simulink model "system_integration_v3"  (R2024a)
settings: Solver=FixedStepDiscrete  StartTime=0.0  StopTime=200  RelTol=1e-3
values from neighbouring files (symbols this model uses):
  Ts = 1/Fs    (= 7.50007500075e-06)    [new_generation_coeff.m]    (also in simon_test.m; simple_fft_test.m = 1/F; testPSD_c2d.m; testPSD_simulink.m)
undefined symbols (not defined in the file or in its folder): magnitude
libraries: hdlsllib x84, embmathops x6, hdlmdlgenlib x1, dsphdlxfrm2 x1
(part 3 of 5)

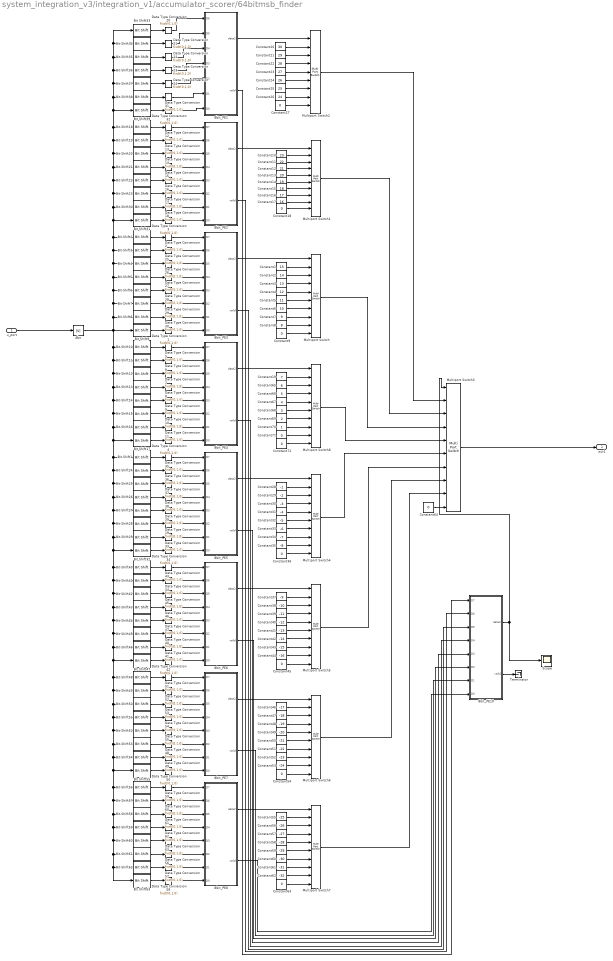
== system system_integration_v3/integration_v1/accumulator_scorer/64bitmsb_finder ==
  u_port : Inport
  8bit_PE1 : Subsystem
  8bit_PE10 : Subsystem
  8bit_PE2 : Subsystem
  8bit_PE3 : Subsystem
  8bit_PE4 : Subsystem
  8bit_PE5 : Subsystem
  8bit_PE6 : Subsystem
  8bit_PE7 : Subsystem
  8bit_PE8 : Subsystem
  Abs : Abs  SaturateOnIntegerOverflow=off
  Bit Shift1 : hdlsllib/Logic and Bit Operations/Bit Shift  mode=Shift Left Logical  N=1
  Bit Shift10 : hdlsllib/Logic and Bit Operations/Bit Shift  mode=Shift Right Logical  N=7
  Bit Shift11 : hdlsllib/Logic and Bit Operations/Bit Shift  mode=Shift Right Logical  N=6
  Bit Shift12 : hdlsllib/Logic and Bit Operations/Bit Shift  mode=Shift Right Logical  N=5
  Bit Shift13 : hdlsllib/Logic and Bit Operations/Bit Shift  mode=Shift Right Logical  N=4
  Bit Shift14 : hdlsllib/Logic and Bit Operations/Bit Shift  mode=Shift Right Logical  N=3
  Bit Shift15 : hdlsllib/Logic and Bit Operations/Bit Shift  mode=Shift Right Logical  N=2
  Bit Shift16 : hdlsllib/Logic and Bit Operations/Bit Shift  mode=Shift Right Logical  N=1
  Bit Shift17 : hdlsllib/Logic and Bit Operations/Bit Shift  mode=Shift Right Logical  N=0
  Bit Shift18 : hdlsllib/Logic and Bit Operations/Bit Shift  mode=Shift Right Logical  N=23
  Bit Shift19 : hdlsllib/Logic and Bit Operations/Bit Shift  mode=Shift Right Logical  N=22
  Bit Shift2 : hdlsllib/Logic and Bit Operations/Bit Shift  mode=Shift Right Logical  N=15
  Bit Shift20 : hdlsllib/Logic and Bit Operations/Bit Shift  mode=Shift Right Logical  N=21
  Bit Shift21 : hdlsllib/Logic and Bit Operations/Bit Shift  mode=Shift Right Logical  N=20
  Bit Shift22 : hdlsllib/Logic and Bit Operations/Bit Shift  mode=Shift Right Logical  N=19
  Bit Shift23 : hdlsllib/Logic and Bit Operations/Bit Shift  mode=Shift Right Logical  N=18
  Bit Shift24 : hdlsllib/Logic and Bit Operations/Bit Shift  mode=Shift Left Logical  N=2
  Bit Shift25 : hdlsllib/Logic and Bit Operations/Bit Shift  mode=Shift Left Logical  N=3
  Bit Shift26 : hdlsllib/Logic and Bit Operations/Bit Shift  mode=Shift Left Logical  N=4
  Bit Shift27 : hdlsllib/Logic and Bit Operations/Bit Shift  mode=Shift Left Logical  N=5
  Bit Shift28 : hdlsllib/Logic and Bit Operations/Bit Shift  mode=Shift Left Logical  N=6
  Bit Shift29 : hdlsllib/Logic and Bit Operations/Bit Shift  mode=Shift Left Logical  N=7
  Bit Shift3 : hdlsllib/Logic and Bit Operations/Bit Shift  mode=Shift Right Logical  N=14
  Bit Shift30 : hdlsllib/Logic and Bit Operations/Bit Shift  mode=Shift Right Logical  N=17
  Bit Shift31 : hdlsllib/Logic and Bit Operations/Bit Shift  mode=Shift Right Logical  N=16
  Bit Shift32 : hdlsllib/Logic and Bit Operations/Bit Shift  mode=Shift Left Logical  N=8
  Bit Shift33 : hdlsllib/Logic and Bit Operations/Bit Shift  mode=Shift Right Logical  N=30
  Bit Shift34 : hdlsllib/Logic and Bit Operations/Bit Shift  mode=Shift Right Logical  N=29
  Bit Shift35 : hdlsllib/Logic and Bit Operations/Bit Shift  mode=Shift Right Logical  N=28
  Bit Shift36 : hdlsllib/Logic and Bit Operations/Bit Shift  mode=Shift Right Logical  N=27
  Bit Shift37 : hdlsllib/Logic and Bit Operations/Bit Shift  mode=Shift Right Logical  N=26
  Bit Shift38 : hdlsllib/Logic and Bit Operations/Bit Shift  mode=Shift Right Logical  N=25
  Bit Shift39 : hdlsllib/Logic and Bit Operations/Bit Shift  mode=Shift Right Logical  N=24
  Bit Shift4 : hdlsllib/Logic and Bit Operations/Bit Shift  mode=Shift Right Logical  N=13
  Bit Shift40 : hdlsllib/Logic and Bit Operations/Bit Shift  mode=Shift Left Logical  N=9
  Bit Shift41 : hdlsllib/Logic and Bit Operations/Bit Shift  mode=Shift Left Logical  N=10
  Bit Shift42 : hdlsllib/Logic and Bit Operations/Bit Shift  mode=Shift Left Logical  N=11
  Bit Shift43 : hdlsllib/Logic and Bit Operations/Bit Shift  mode=Shift Left Logical  N=12
  Bit Shift44 : hdlsllib/Logic and Bit Operations/Bit Shift  mode=Shift Left Logical  N=13
  Bit Shift45 : hdlsllib/Logic and Bit Operations/Bit Shift  mode=Shift Left Logical  N=14
  Bit Shift46 : hdlsllib/Logic and Bit Operations/Bit Shift  mode=Shift Left Logical  N=15
  Bit Shift47 : hdlsllib/Logic and Bit Operations/Bit Shift  mode=Shift Left Logical  N=16
  Bit Shift48 : hdlsllib/Logic and Bit Operations/Bit Shift  mode=Shift Left Logical  N=17
  Bit Shift49 : hdlsllib/Logic and Bit Operations/Bit Shift  mode=Shift Left Logical  N=18
  Bit Shift5 : hdlsllib/Logic and Bit Operations/Bit Shift  mode=Shift Right Logical  N=12
  Bit Shift50 : hdlsllib/Logic and Bit Operations/Bit Shift  mode=Shift Left Logical  N=19
  Bit Shift51 : hdlsllib/Logic and Bit Operations/Bit Shift  mode=Shift Left Logical  N=20
  Bit Shift52 : hdlsllib/Logic and Bit Operations/Bit Shift  mode=Shift Left Logical  N=21
  Bit Shift53 : hdlsllib/Logic and Bit Operations/Bit Shift  mode=Shift Left Logical  N=22
  Bit Shift54 : hdlsllib/Logic and Bit Operations/Bit Shift  mode=Shift Left Logical  N=23
  Bit Shift55 : hdlsllib/Logic and Bit Operations/Bit Shift  mode=Shift Left Logical  N=24
  Bit Shift56 : hdlsllib/Logic and Bit Operations/Bit Shift  mode=Shift Left Logical  N=25
  Bit Shift57 : hdlsllib/Logic and Bit Operations/Bit Shift  mode=Shift Left Logical  N=26
  Bit Shift58 : hdlsllib/Logic and Bit Operations/Bit Shift  mode=Shift Left Logical  N=27
  Bit Shift59 : hdlsllib/Logic and Bit Operations/Bit Shift  mode=Shift Left Logical  N=28
  Bit Shift6 : hdlsllib/Logic and Bit Operations/Bit Shift  mode=Shift Right Logical  N=11
  Bit Shift60 : hdlsllib/Logic and Bit Operations/Bit Shift  mode=Shift Left Logical  N=29
  Bit Shift61 : hdlsllib/Logic and Bit Operations/Bit Shift  mode=Shift Left Logical  N=30
  Bit Shift62 : hdlsllib/Logic and Bit Operations/Bit Shift  mode=Shift Left Logical  N=31
  Bit Shift63 : hdlsllib/Logic and Bit Operations/Bit Shift  mode=Shift Left Logical  N=32
  Bit Shift7 : hdlsllib/Logic and Bit Operations/Bit Shift  mode=Shift Right Logical  N=10
  Bit Shift8 : hdlsllib/Logic and Bit Operations/Bit Shift  mode=Shift Right Logical  N=9
  Bit Shift9 : hdlsllib/Logic and Bit Operations/Bit Shift  mode=Shift Right Logical  N=8
  Constant1 : Constant  Value=15  OutDataTypeStr=fixdt(1,64,32)  SampleTime=Ts
  Constant10 : Constant  Value=23  OutDataTypeStr=fixdt(1,64,32)  SampleTime=Ts
  Constant11 : Constant  Value=22  OutDataTypeStr=fixdt(1,64,32)  SampleTime=Ts
  Constant12 : Constant  Value=21  OutDataTypeStr=fixdt(1,64,32)  SampleTime=Ts
  Constant13 : Constant  Value=20  OutDataTypeStr=fixdt(1,64,32)  SampleTime=Ts
  Constant14 : Constant  Value=19  OutDataTypeStr=fixdt(1,64,32)  SampleTime=Ts
  Constant15 : Constant  Value=18  OutDataTypeStr=fixdt(1,64,32)  SampleTime=Ts
  Constant16 : Constant  Value=17  OutDataTypeStr=fixdt(1,64,32)  SampleTime=Ts
  Constant17 : Constant  Value=16  OutDataTypeStr=fixdt(1,64,32)  SampleTime=Ts
  Constant{9,18,27,36,45,54,63..64,71..72} (10 alike) : Constant  Value=0  OutDataTypeStr=fixdt(1,64,32)  SampleTime=Ts
  Constant19 : Constant  Value=7  OutDataTypeStr=fixdt(1,64,32)  SampleTime=Ts
  Constant2 : Constant  Value=14  OutDataTypeStr=fixdt(1,64,32)  SampleTime=Ts
  Constant20 : Constant  Value=30  OutDataTypeStr=fixdt(1,64,32)  SampleTime=Ts
  Constant21 : Constant  Value=29  OutDataTypeStr=fixdt(1,64,32)  SampleTime=Ts
  Constant22 : Constant  Value=28  OutDataTypeStr=fixdt(1,64,32)  SampleTime=Ts
  Constant23 : Constant  Value=27  OutDataTypeStr=fixdt(1,64,32)  SampleTime=Ts
  Constant24 : Constant  Value=26  OutDataTypeStr=fixdt(1,64,32)  SampleTime=Ts
  Constant25 : Constant  Value=25  OutDataTypeStr=fixdt(1,64,32)  SampleTime=Ts
  Constant26 : Constant  Value=24  OutDataTypeStr=fixdt(1,64,32)  SampleTime=Ts
  Constant28 : Constant  Value=-1  OutDataTypeStr=fixdt(1,64,32)  SampleTime=Ts
  Constant29 : Constant  Value=-2  OutDataTypeStr=fixdt(1,64,32)  SampleTime=Ts
  Constant3 : Constant  Value=13  OutDataTypeStr=fixdt(1,64,32)  SampleTime=Ts
  Constant30 : Constant  Value=-3  OutDataTypeStr=fixdt(1,64,32)  SampleTime=Ts
  Constant31 : Constant  Value=-4  OutDataTypeStr=fixdt(1,64,32)  SampleTime=Ts
  Constant32 : Constant  Value=-5  OutDataTypeStr=fixdt(1,64,32)  SampleTime=Ts
  Constant33 : Constant  Value=-6  OutDataTypeStr=fixdt(1,64,32)  SampleTime=Ts
  Constant34 : Constant  Value=-7  OutDataTypeStr=fixdt(1,64,32)  SampleTime=Ts
  Constant35 : Constant  Value=-8  OutDataTypeStr=fixdt(1,64,32)  SampleTime=Ts
  Constant37 : Constant  Value=-9  OutDataTypeStr=fixdt(1,64,32)  SampleTime=Ts
  Constant38 : Constant  Value=-10  OutDataTypeStr=fixdt(1,64,32)  SampleTime=Ts
  Constant39 : Constant  Value=-11  OutDataTypeStr=fixdt(1,64,32)  SampleTime=Ts
  Constant4 : Constant  Value=12  OutDataTypeStr=fixdt(1,64,32)  SampleTime=Ts
  Constant40 : Constant  Value=-12  OutDataTypeStr=fixdt(1,64,32)  SampleTime=Ts
  Constant41 : Constant  Value=-13  OutDataTypeStr=fixdt(1,64,32)  SampleTime=Ts
  Constant42 : Constant  Value=-14  OutDataTypeStr=fixdt(1,64,32)  SampleTime=Ts
  Constant43 : Constant  Value=-15  OutDataTypeStr=fixdt(1,64,32)  SampleTime=Ts
  Constant44 : Constant  Value=-16  OutDataTypeStr=fixdt(1,64,32)  SampleTime=Ts
  Constant46 : Constant  Value=-17  OutDataTypeStr=fixdt(1,64,32)  SampleTime=Ts
  Constant47 : Constant  Value=-18  OutDataTypeStr=fixdt(1,64,32)  SampleTime=Ts
  Constant48 : Constant  Value=-19  OutDataTypeStr=fixdt(1,64,32)  SampleTime=Ts
  Constant49 : Constant  Value=-20  OutDataTypeStr=fixdt(1,64,32)  SampleTime=Ts
  Constant5 : Constant  Value=11  OutDataTypeStr=fixdt(1,64,32)  SampleTime=Ts
  Constant50 : Constant  Value=-21  OutDataTypeStr=fixdt(1,64,32)  SampleTime=Ts
  Constant51 : Constant  Value=-22  OutDataTypeStr=fixdt(1,64,32)  SampleTime=Ts
  Constant52 : Constant  Value=-23  OutDataTypeStr=fixdt(1,64,32)  SampleTime=Ts
  Constant53 : Constant  Value=-24  OutDataTypeStr=fixdt(1,64,32)  SampleTime=Ts
  Constant55 : Constant  Value=-25  OutDataTypeStr=fixdt(1,64,32)  SampleTime=Ts
  Constant56 : Constant  Value=-26  OutDataTypeStr=fixdt(1,64,32)  SampleTime=Ts
  Constant57 : Constant  Value=-27  OutDataTypeStr=fixdt(1,64,32)  SampleTime=Ts
  Constant58 : Constant  Value=-28  OutDataTypeStr=fixdt(1,64,32)  SampleTime=Ts
  Constant59 : Constant  Value=-29  OutDataTypeStr=fixdt(1,64,32)  SampleTime=Ts
  Constant6 : Constant  Value=10  OutDataTypeStr=fixdt(1,64,32)  SampleTime=Ts
  Constant60 : Constant  Value=-30  OutDataTypeStr=fixdt(1,64,32)  SampleTime=Ts
  Constant61 : Constant  Value=-31  OutDataTypeStr=fixdt(1,64,32)  SampleTime=Ts
  Constant62 : Constant  Value=-32  OutDataTypeStr=fixdt(1,64,32)  SampleTime=Ts
  Constant65 : Constant  Value=6  OutDataTypeStr=fixdt(1,64,32)  SampleTime=Ts
  Constant66 : Constant  Value=5  OutDataTypeStr=fixdt(1,64,32)  SampleTime=Ts
  Constant67 : Constant  Value=4  OutDataTypeStr=fixdt(1,64,32)  SampleTime=Ts
  Constant68 : Constant  Value=3  OutDataTypeStr=fixdt(1,64,32)  SampleTime=Ts
  Constant69 : Constant  Value=2  OutDataTypeStr=fixdt(1,64,32)  SampleTime=Ts
  Constant7 : Constant  Value=9  OutDataTypeStr=fixdt(1,64,32)  SampleTime=Ts
  Constant70 : Constant  OutDataTypeStr=fixdt(1,64,32)  SampleTime=Ts
  Constant8 : Constant  Value=8  OutDataTypeStr=fixdt(1,64,32)  SampleTime=Ts
  Data Type Conversion{1..63} (63 alike) : DataTypeConversion  OutDataTypeStr=fixdt(0,1,0)  SaturateOnIntegerOverflow=off  RndMeth=Floor
  Multiport Switch{,1,4..8} (7 alike) : MultiPortSwitch  DataPortOrder=Specify indices  Inputs=8  DataPortIndices={8,7,6,5,4,3,2,1}  DataPortForDefault=Additional data port  DiagnosticForDefault=None  SaturateOnIntegerOverflow=off  InputSameDT=off
  Multiport Switch2 : MultiPortSwitch  DataPortOrder=Specify indices  Inputs=8  DataPortIndices={7,6,5,4,3,2,1}  DataPortForDefault=Additional data port  DiagnosticForDefault=None  SaturateOnIntegerOverflow=off  InputSameDT=off
  Multiport Switch3 : MultiPortSwitch  DataPortOrder=Specify indices  Inputs=8  DataPortIndices={8, 7, 6, 5, 4,3,2,1}  DataPortForDefault=Additional data port  DiagnosticForDefault=None  SaturateOnIntegerOverflow=off  InputSameDT=off
  Scope : Scope
  Terminator : Terminator
  out1 : Outport
  wires:
  Data Type Conversion16/1 -> 8bit_PE2/5(D3)
  Bit Shift19/1 -> Data Type Conversion13/1
  Bit Shift22/1 -> Data Type Conversion16/1
  Constant5/1 -> Multiport Switch/6
  8bit_PE4/1(data2) -> Multiport Switch8/1
  Data Type Conversion17/1 -> 8bit_PE2/6(D2)
  Multiport Switch3/1 -> out1/1
  Constant6/1 -> Multiport Switch/7
  8bit_PE10/1(data2) -> Multiport Switch3/1, Scope/1
  Data Type Conversion29/1 -> 8bit_PE3/6(D2)
  Bit Shift11/1 -> Data Type Conversion6/1
  Bit Shift7/1 -> Data Type Conversion29/1
  Data Type Conversion28/1 -> 8bit_PE3/5(D3)
  Constant23/1 -> Multiport Switch2/5
  Bit Shift3/1 -> Data Type Conversion25/1
  Constant10/1 -> Multiport Switch1/2
  Data Type Conversion26/1 -> 8bit_PE3/3(D5)
  Bit Shift8/1 -> Data Type Conversion30/1
  Data Type Conversion27/1 -> 8bit_PE3/4(D4)
  Data Type Conversion12/1 -> 8bit_PE2/1(D7)
  Data Type Conversion18/1 -> 8bit_PE2/7(D1)
  Bit Shift4/1 -> Data Type Conversion26/1
  Data Type Conversion25/1 -> 8bit_PE3/2(D6)
  Data Type Conversion13/1 -> 8bit_PE2/2(D6)
  Data Type Conversion7/1 -> 8bit_PE4/3(D5)
  Bit Shift5/1 -> Data Type Conversion27/1
  Data Type Conversion30/1 -> 8bit_PE3/7(D1)
  Bit Shift38/1 -> Data Type Conversion31/1
  Data Type Conversion14/1 -> 8bit_PE2/3(D5)
  8bit_PE2/1(data2) -> Multiport Switch1/1
  Bit Shift13/1 -> Data Type Conversion8/1
  8bit_PE1/1(data2) -> Multiport Switch2/1
  Bit Shift2/1 -> Data Type Conversion2/1
  Data Type Conversion5/1 -> 8bit_PE4/1(D7)
  Data Type Conversion8/1 -> 8bit_PE4/4(D4)
  Bit Shift21/1 -> Data Type Conversion15/1
  Bit Shift10/1 -> Data Type Conversion5/1
  Bit Shift30/1 -> Data Type Conversion18/1
  Data Type Conversion15/1 -> 8bit_PE2/4(D4)
  Data Type Conversion23/1 -> 8bit_PE1/4(D3)
  Data Type Conversion6/1 -> 8bit_PE4/2(D6)
  Data Type Conversion1/1 -> 8bit_PE3/8(D0)
  Constant9/1 -> Multiport Switch/10
  Bit Shift14/1 -> Data Type Conversion9/1
  Data Type Conversion4/1 -> 8bit_PE4/8(D0)
  Data Type Conversion31/1 -> 8bit_PE1/6(D1)
  Bit Shift15/1 -> Data Type Conversion10/1
  Bit Shift18/1 -> Data Type Conversion12/1
  Data Type Conversion10/1 -> 8bit_PE4/6(D2)
  Bit Shift37/1 -> Data Type Conversion24/1
  Constant2/1 -> Multiport Switch/3
  Constant3/1 -> Multiport Switch/4
  Bit Shift36/1 -> Data Type Conversion23/1
  Bit Shift23/1 -> Data Type Conversion17/1
  Constant16/1 -> Multiport Switch1/8
  Constant25/1 -> Multiport Switch2/7
  Constant1/1 -> Multiport Switch/2
  Bit Shift34/1 -> Data Type Conversion21/1
  Data Type Conversion22/1 -> 8bit_PE1/3(D4)
  Multiport Switch2/1 -> Multiport Switch3/2
  Bit Shift33/1 -> Data Type Conversion20/1
  Bit Shift31/1 -> Data Type Conversion3/1
  Bit Shift39/1 -> Data Type Conversion32/1
  Data Type Conversion11/1 -> 8bit_PE4/7(D1)
  Bit Shift35/1 -> Data Type Conversion22/1
  Constant7/1 -> Multiport Switch/8
  Bit Shift9/1 -> Data Type Conversion1/1
  Constant4/1 -> Multiport Switch/5
  Bit Shift20/1 -> Data Type Conversion14/1
  Data Type Conversion24/1 -> 8bit_PE1/5(D2)
  Constant12/1 -> Multiport Switch1/4
  Constant8/1 -> Multiport Switch/9
  Constant21/1 -> Multiport Switch2/3
  Constant15/1 -> Multiport Switch1/7
  Data Type Conversion9/1 -> 8bit_PE4/5(D3)
  Constant13/1 -> Multiport Switch1/5
  Multiport Switch1/1 -> Multiport Switch3/3
  Constant14/1 -> Multiport Switch1/6
  Multiport Switch/1 -> Multiport Switch3/4
  Data Type Conversion21/1 -> 8bit_PE1/2(D5)
  Constant20/1 -> Multiport Switch2/2
  Constant18/1 -> Multiport Switch1/10
  Constant24/1 -> Multiport Switch2/6
  Constant22/1 -> Multiport Switch2/4
  Constant11/1 -> Multiport Switch1/3
  Constant27/1 -> Multiport Switch2/9
  8bit_PE3/1(data2) -> Multiport Switch/1
  Bit Shift6/1 -> Data Type Conversion28/1
  Constant17/1 -> Multiport Switch1/9
  Data Type Conversion20/1 -> 8bit_PE1/1(D6)
  Data Type Conversion32/1 -> 8bit_PE1/7(D0)
  Data Type Conversion3/1 -> 8bit_PE2/8(D0)
  Bit Shift12/1 -> Data Type Conversion7/1
  Data Type Conversion2/1 -> 8bit_PE3/1(D7)
  Bit Shift16/1 -> Data Type Conversion11/1
  Bit Shift17/1 -> Data Type Conversion4/1
  Constant26/1 -> Multiport Switch2/8
  u_port/1 -> Abs/1
  Bit Shift32/1 -> Data Type Conversion34/1
  Bit Shift29/1 -> Data Type Conversion33/1
  Bit Shift25/1 -> Data Type Conversion37/1
  Data Type Conversion39/1 -> 8bit_PE5/5(D3)
  Data Type Conversion33/1 -> 8bit_PE5/7(D1)
  Data Type Conversion19/1 -> 8bit_PE5/6(D2)
  Bit Shift28/1 -> Data Type Conversion19/1
  Data Type Conversion34/1 -> 8bit_PE5/8(D0)
  Bit Shift27/1 -> Data Type Conversion39/1
  Data Type Conversion36/1 -> 8bit_PE5/2(D6)
  Bit Shift1/1 -> Data Type Conversion35/1
  Data Type Conversion38/1 -> 8bit_PE5/4(D4)
  Data Type Conversion35/1 -> 8bit_PE5/1(D7)
  Bit Shift26/1 -> Data Type Conversion38/1
  Data Type Conversion37/1 -> 8bit_PE5/3(D5)
  Bit Shift24/1 -> Data Type Conversion36/1
  Bit Shift41/1 -> Data Type Conversion44/1
  Data Type Conversion45/1 -> 8bit_PE6/3(D5)
  Bit Shift43/1 -> Data Type Conversion46/1
  Data Type Conversion43/1 -> 8bit_PE6/1(D7)
  Data Type Conversion46/1 -> 8bit_PE6/4(D4)
  Bit Shift40/1 -> Data Type Conversion43/1
  Data Type Conversion44/1 -> 8bit_PE6/2(D6)
  Bit Shift44/1 -> Data Type Conversion47/1
  Data Type Conversion42/1 -> 8bit_PE6/8(D0)
  Bit Shift45/1 -> Data Type Conversion40/1
  Data Type Conversion40/1 -> 8bit_PE6/6(D2)
  Data Type Conversion41/1 -> 8bit_PE6/7(D1)
  Data Type Conversion47/1 -> 8bit_PE6/5(D3)
  Bit Shift42/1 -> Data Type Conversion45/1
  Bit Shift46/1 -> Data Type Conversion41/1
  Bit Shift47/1 -> Data Type Conversion42/1
  Bit Shift55/1 -> Data Type Conversion50/1
  Bit Shift54/1 -> Data Type Conversion49/1
  Bit Shift50/1 -> Data Type Conversion53/1
  Data Type Conversion55/1 -> 8bit_PE7/5(D3)
  Data Type Conversion49/1 -> 8bit_PE7/7(D1)
  Data Type Conversion48/1 -> 8bit_PE7/6(D2)
  Bit Shift53/1 -> Data Type Conversion48/1
  Data Type Conversion50/1 -> 8bit_PE7/8(D0)
  Bit Shift52/1 -> Data Type Conversion55/1
  Data Type Conversion52/1 -> 8bit_PE7/2(D6)
  Bit Shift48/1 -> Data Type Conversion51/1
  Data Type Conversion54/1 -> 8bit_PE7/4(D4)
  Data Type Conversion51/1 -> 8bit_PE7/1(D7)
  Bit Shift51/1 -> Data Type Conversion54/1
  Data Type Conversion53/1 -> 8bit_PE7/3(D5)
  Bit Shift49/1 -> Data Type Conversion52/1
  Abs/1 -> Bit Shift23/1, Bit Shift22/1, Bit Shift21/1, Bit Shift20/1, Bit Shift19/1, Bit Shift37/1, Bit Shift36/1, Bit Shift33/1, Bit Shift34/1, Bit Shift35/1, Bit Shift38/1, Bit Shift39/1, Bit Shift18/1, Bit Shift30/1, Bit Shift31/1, Bit Shift2/1, Bit Shift3/1, Bit Shift4/1, Bit Shift5/1, Bit Shift6/1, Bit Shift7/1, Bit Shift8/1, Bit Shift11/1, Bit Shift12/1, Bit Shift13/1, Bit Shift14/1, Bit Shift15/1, Bit Shift16/1, Bit Shift17/1, Bit Shift1/1, Bit Shift41/1, Bit Shift42/1, Bit Shift43/1, Bit Shift44/1, Bit Shift45/1, Bit Shift46/1, Bit Shift63/1, Bit Shift62/1, Bit Shift61/1, Bit Shift60/1, Bit Shift59/1, Bit Shift58/1, Bit Shift57/1, Bit Shift56/1, Bit Shift55/1, Bit Shift54/1, Bit Shift53/1, Bit Shift52/1, Bit Shift51/1, Bit Shift50/1, Bit Shift49/1, Bit Shift48/1, Bit Shift47/1, Bit Shift40/1, Bit Shift32/1, Bit Shift29/1, Bit Shift28/1, Bit Shift27/1, Bit Shift26/1, Bit Shift25/1, Bit Shift24/1, Bit Shift10/1, Bit Shift9/1
  Bit Shift57/1 -> Data Type Conversion60/1
  Data Type Conversion61/1 -> 8bit_PE8/3(D5)
  Bit Shift59/1 -> Data Type Conversion62/1
  Data Type Conversion59/1 -> 8bit_PE8/1(D7)
  Data Type Conversion62/1 -> 8bit_PE8/4(D4)
  Bit Shift56/1 -> Data Type Conversion59/1
  Data Type Conversion60/1 -> 8bit_PE8/2(D6)
  Bit Shift60/1 -> Data Type Conversion63/1
  Data Type Conversion58/1 -> 8bit_PE8/8(D0)
  Bit Shift61/1 -> Data Type Conversion56/1
  Data Type Conversion56/1 -> 8bit_PE8/6(D2)
  Data Type Conversion57/1 -> 8bit_PE8/7(D1)
  Data Type Conversion63/1 -> 8bit_PE8/5(D3)
  Bit Shift58/1 -> Data Type Conversion61/1
  Bit Shift62/1 -> Data Type Conversion57/1
  Bit Shift63/1 -> Data Type Conversion58/1
  8bit_PE5/1(data2) -> Multiport Switch4/1
  Constant35/1 -> Multiport Switch4/9
  Constant31/1 -> Multiport Switch4/5
  Constant34/1 -> Multiport Switch4/8
  Constant28/1 -> Multiport Switch4/2
  Constant30/1 -> Multiport Switch4/4
  Constant29/1 -> Multiport Switch4/3
  Constant36/1 -> Multiport Switch4/10
  Constant33/1 -> Multiport Switch4/7
  Constant32/1 -> Multiport Switch4/6
  Constant41/1 -> Multiport Switch5/6
  Constant42/1 -> Multiport Switch5/7
  Constant45/1 -> Multiport Switch5/10
  Constant38/1 -> Multiport Switch5/3
  Constant39/1 -> Multiport Switch5/4
  Constant37/1 -> Multiport Switch5/2
  Constant43/1 -> Multiport Switch5/8
  Constant40/1 -> Multiport Switch5/5
  Constant44/1 -> Multiport Switch5/9
  8bit_PE6/1(data2) -> Multiport Switch5/1
  8bit_PE7/1(data2) -> Multiport Switch6/1
  Constant53/1 -> Multiport Switch6/9
  Constant49/1 -> Multiport Switch6/5
  Constant52/1 -> Multiport Switch6/8
  Constant46/1 -> Multiport Switch6/2
  Constant48/1 -> Multiport Switch6/4
  Constant47/1 -> Multiport Switch6/3
  Constant54/1 -> Multiport Switch6/10
  Constant51/1 -> Multiport Switch6/7
  Constant50/1 -> Multiport Switch6/6
  Constant59/1 -> Multiport Switch7/6
  Constant60/1 -> Multiport Switch7/7
  Constant63/1 -> Multiport Switch7/10
  Constant56/1 -> Multiport Switch7/3
  Constant57/1 -> Multiport Switch7/4
  Constant55/1 -> Multiport Switch7/2
  Constant61/1 -> Multiport Switch7/8
  Constant58/1 -> Multiport Switch7/5
  Constant62/1 -> Multiport Switch7/9
  8bit_PE8/1(data2) -> Multiport Switch7/1
  Multiport Switch4/1 -> Multiport Switch3/6
  Multiport Switch5/1 -> Multiport Switch3/7
  Multiport Switch6/1 -> Multiport Switch3/8
  Multiport Switch7/1 -> Multiport Switch3/9
  8bit_PE1/2(valid) -> 8bit_PE10/1(D7)
  8bit_PE2/2(valid) -> 8bit_PE10/2(D6)
  8bit_PE4/2(valid) -> 8bit_PE10/4(D4)
  8bit_PE5/2(valid) -> 8bit_PE10/5(D3)
  8bit_PE6/2(valid) -> 8bit_PE10/6(D2)
  8bit_PE7/2(valid) -> 8bit_PE10/7(D1)
  8bit_PE8/2(valid) -> 8bit_PE10/8(D0)
  8bit_PE3/2(valid) -> 8bit_PE10/3(D5)
  Constant64/1 -> Multiport Switch3/10
  Constant71/1 -> Multiport Switch8/9
  Constant67/1 -> Multiport Switch8/5
  Constant70/1 -> Multiport Switch8/8
  Constant19/1 -> Multiport Switch8/2
  Constant66/1 -> Multiport Switch8/4
  Constant65/1 -> Multiport Switch8/3
  Constant72/1 -> Multiport Switch8/10
  Constant69/1 -> Multiport Switch8/7
  Constant68/1 -> Multiport Switch8/6
  Multiport Switch8/1 -> Multiport Switch3/5
  8bit_PE10/2(valid) -> Terminator/1

== system system_integration_v3/integration_v1/D2/individual1/Subsystem ==
  reg_in : Inport
  enable : Inport  Port=2
  Delay : Delay  DelayLength=1  InitialCondition=0  SampleTime=Ts
  Switch : Switch  Criteria=u2 > Threshold  SaturateOnIntegerOverflow=off  InputSameDT=off
  reg_out : Outport
  wires:
  Delay/1 -> reg_out/1, Switch/3
  Switch/1 -> Delay/1
  enable/1 -> Switch/2
  reg_in/1 -> Switch/1

== system system_integration_v3/integration_v1/D2/individual1/Subsystem1 ==
  reg_in : Inport
  enable : Inport  Port=2
  Delay : Delay  DelayLength=1  InitialCondition=0  SampleTime=Ts
  Switch : Switch  Criteria=u2 > Threshold  SaturateOnIntegerOverflow=off  InputSameDT=off
  reg_out : Outport
  wires:
  Delay/1 -> reg_out/1, Switch/3
  Switch/1 -> Delay/1
  enable/1 -> Switch/2
  reg_in/1 -> Switch/1

== system system_integration_v3/integration_v1/D2/individual1/Subsystem2 ==
  reg_in : Inport
  enable : Inport  Port=2
  Delay : Delay  DelayLength=1  InitialCondition=0  SampleTime=Ts
  Switch : Switch  Criteria=u2 > Threshold  SaturateOnIntegerOverflow=off  InputSameDT=off
  reg_out : Outport
  wires:
  Delay/1 -> reg_out/1, Switch/3
  Switch/1 -> Delay/1
  enable/1 -> Switch/2
  reg_in/1 -> Switch/1

== system system_integration_v3/integration_v1/D2/individual1/Subsystem3 ==
  reg_in : Inport
  enable : Inport  Port=2
  Delay : Delay  DelayLength=1  InitialCondition=0  SampleTime=Ts
  Switch : Switch  Criteria=u2 > Threshold  SaturateOnIntegerOverflow=off  InputSameDT=off
  reg_out : Outport
  wires:
  Delay/1 -> reg_out/1, Switch/3
  Switch/1 -> Delay/1
  enable/1 -> Switch/2
  reg_in/1 -> Switch/1

== system system_integration_v3/integration_v1/D2/individual1/Subsystem4 ==
  reg_in : Inport
  enable : Inport  Port=2
  Delay : Delay  DelayLength=1  InitialCondition=0  SampleTime=Ts
  Switch : Switch  Criteria=u2 > Threshold  SaturateOnIntegerOverflow=off  InputSameDT=off
  reg_out : Outport
  wires:
  Delay/1 -> reg_out/1, Switch/3
  Switch/1 -> Delay/1
  enable/1 -> Switch/2
  reg_in/1 -> Switch/1

== system system_integration_v3/integration_v1/D2/individual1/Subsystem5 ==
  reg_in : Inport
  enable : Inport  Port=2
  Delay : Delay  DelayLength=1  InitialCondition=0  SampleTime=Ts
  Switch : Switch  Criteria=u2 > Threshold  SaturateOnIntegerOverflow=off  InputSameDT=off
  reg_out : Outport
  wires:
  Delay/1 -> reg_out/1, Switch/3
  Switch/1 -> Delay/1
  enable/1 -> Switch/2
  reg_in/1 -> Switch/1

== system system_integration_v3/integration_v1/D2/individual1/Subsystem6 ==
  reg_in : Inport
  enable : Inport  Port=2
  Delay : Delay  DelayLength=1  InitialCondition=0  SampleTime=Ts
  Switch : Switch  Criteria=u2 > Threshold  SaturateOnIntegerOverflow=off  InputSameDT=off
  reg_out : Outport
  wires:
  reg_in/1 -> Switch/1
  enable/1 -> Switch/2
  Switch/1 -> Delay/1
  Delay/1 -> Switch/3, reg_out/1

== system system_integration_v3/integration_v1/GA_main/coefficent_array/individual1 ==
  reg_in : Inport
  reg_in1 : Inport  Port=2
  reg_in2 : Inport  Port=3
  reg_in3 : Inport  Port=4
  reg_in4 : Inport  Port=5
  reg_in5 : Inport  Port=6
  reg_in6 : Inport  Port=7
  enable : Inport  Port=8
  Subsystem : Subsystem
  Subsystem1 : Subsystem
  Subsystem2 : Subsystem
  Subsystem3 : Subsystem
  Subsystem4 : Subsystem
  Subsystem5 : Subsystem
  Subsystem6 : Subsystem
  score : Outport
  a2 : Outport  Port=2
  a3 : Outport  Port=3
  a4 : Outport  Port=4
  b2 : Outport  Port=5
  b3 : Outport  Port=6
  b4 : Outport  Port=7
  wires:
  enable/1 -> Subsystem3/2(enable), Subsystem4/2(enable), Subsystem5/2(enable), Subsystem6/2(enable), Subsystem2/2(enable), Subsystem1/2(enable), Subsystem/2(enable)
  Subsystem2/1(reg_out) -> a3/1
  Subsystem4/1(reg_out) -> b2/1
  Subsystem3/1(reg_out) -> a4/1
  Subsystem1/1(reg_out) -> a2/1
  reg_in/1 -> Subsystem/1(reg_in)
  Subsystem/1(reg_out) -> score/1
  reg_in1/1 -> Subsystem1/1(reg_in)
  reg_in2/1 -> Subsystem2/1(reg_in)
  reg_in3/1 -> Subsystem3/1(reg_in)
  Subsystem5/1(reg_out) -> b3/1
  reg_in4/1 -> Subsystem4/1(reg_in)
  reg_in5/1 -> Subsystem5/1(reg_in)
  Subsystem6/1(reg_out) -> b4/1
  reg_in6/1 -> Subsystem6/1(reg_in)

== system system_integration_v3/integration_v1/GA_main/coefficent_array/individual2 ==
  reg_in : Inport
  reg_in1 : Inport  Port=2
  reg_in2 : Inport  Port=3
  reg_in3 : Inport  Port=4
  reg_in4 : Inport  Port=5
  reg_in5 : Inport  Port=6
  reg_in6 : Inport  Port=7
  enable : Inport  Port=8
  Subsystem : Subsystem
  Subsystem1 : Subsystem
  Subsystem2 : Subsystem
  Subsystem3 : Subsystem
  Subsystem4 : Subsystem
  Subsystem5 : Subsystem
  Subsystem6 : Subsystem
  score : Outport
  a2 : Outport  Port=2
  a3 : Outport  Port=3
  a4 : Outport  Port=4
  b2 : Outport  Port=5
  b3 : Outport  Port=6
  b4 : Outport  Port=7
  wires:
  reg_in6/1 -> Subsystem6/1(reg_in)
  Subsystem6/1(reg_out) -> b4/1
  reg_in5/1 -> Subsystem5/1(reg_in)
  reg_in4/1 -> Subsystem4/1(reg_in)
  Subsystem5/1(reg_out) -> b3/1
  reg_in3/1 -> Subsystem3/1(reg_in)
  reg_in2/1 -> Subsystem2/1(reg_in)
  reg_in1/1 -> Subsystem1/1(reg_in)
  Subsystem/1(reg_out) -> score/1
  reg_in/1 -> Subsystem/1(reg_in)
  Subsystem1/1(reg_out) -> a2/1
  Subsystem3/1(reg_out) -> a4/1
  Subsystem4/1(reg_out) -> b2/1
  Subsystem2/1(reg_out) -> a3/1
  enable/1 -> Subsystem/2(enable), Subsystem1/2(enable), Subsystem2/2(enable), Subsystem6/2(enable), Subsystem5/2(enable), Subsystem4/2(enable), Subsystem3/2(enable)

== system system_integration_v3/integration_v1/GA_main/coefficent_array/individual3 ==
  reg_in : Inport
  reg_in1 : Inport  Port=2
  reg_in2 : Inport  Port=3
  reg_in3 : Inport  Port=4
  reg_in4 : Inport  Port=5
  reg_in5 : Inport  Port=6
  reg_in6 : Inport  Port=7
  enable : Inport  Port=8
  Subsystem : Subsystem
  Subsystem1 : Subsystem
  Subsystem2 : Subsystem
  Subsystem3 : Subsystem
  Subsystem4 : Subsystem
  Subsystem5 : Subsystem
  Subsystem6 : Subsystem
  score : Outport
  a2 : Outport  Port=2
  a3 : Outport  Port=3
  a4 : Outport  Port=4
  b2 : Outport  Port=5
  b3 : Outport  Port=6
  b4 : Outport  Port=7
  wires:
  enable/1 -> Subsystem3/2(enable), Subsystem4/2(enable), Subsystem5/2(enable), Subsystem6/2(enable), Subsystem2/2(enable), Subsystem1/2(enable), Subsystem/2(enable)
  Subsystem2/1(reg_out) -> a3/1
  Subsystem4/1(reg_out) -> b2/1
  Subsystem3/1(reg_out) -> a4/1
  Subsystem1/1(reg_out) -> a2/1
  reg_in/1 -> Subsystem/1(reg_in)
  Subsystem/1(reg_out) -> score/1
  reg_in1/1 -> Subsystem1/1(reg_in)
  reg_in2/1 -> Subsystem2/1(reg_in)
  reg_in3/1 -> Subsystem3/1(reg_in)
  Subsystem5/1(reg_out) -> b3/1
  reg_in4/1 -> Subsystem4/1(reg_in)
  reg_in5/1 -> Subsystem5/1(reg_in)
  Subsystem6/1(reg_out) -> b4/1
  reg_in6/1 -> Subsystem6/1(reg_in)

== system system_integration_v3/integration_v1/GA_main/coefficent_array/individual4 ==
  reg_in : Inport
  reg_in1 : Inport  Port=2
  reg_in2 : Inport  Port=3
  reg_in3 : Inport  Port=4
  reg_in4 : Inport  Port=5
  reg_in5 : Inport  Port=6
  reg_in6 : Inport  Port=7
  enable : Inport  Port=8
  Subsystem : Subsystem
  Subsystem1 : Subsystem
  Subsystem2 : Subsystem
  Subsystem3 : Subsystem
  Subsystem4 : Subsystem
  Subsystem5 : Subsystem
  Subsystem6 : Subsystem
  score : Outport
  a2 : Outport  Port=2
  a3 : Outport  Port=3
  a4 : Outport  Port=4
  b2 : Outport  Port=5
  b3 : Outport  Port=6
  b4 : Outport  Port=7
  wires:
  reg_in6/1 -> Subsystem6/1(reg_in)
  Subsystem6/1(reg_out) -> b4/1
  reg_in5/1 -> Subsystem5/1(reg_in)
  reg_in4/1 -> Subsystem4/1(reg_in)
  Subsystem5/1(reg_out) -> b3/1
  reg_in3/1 -> Subsystem3/1(reg_in)
  reg_in2/1 -> Subsystem2/1(reg_in)
  reg_in1/1 -> Subsystem1/1(reg_in)
  Subsystem/1(reg_out) -> score/1
  reg_in/1 -> Subsystem/1(reg_in)
  Subsystem1/1(reg_out) -> a2/1
  Subsystem3/1(reg_out) -> a4/1
  Subsystem4/1(reg_out) -> b2/1
  Subsystem2/1(reg_out) -> a3/1
  enable/1 -> Subsystem/2(enable), Subsystem1/2(enable), Subsystem2/2(enable), Subsystem6/2(enable), Subsystem5/2(enable), Subsystem4/2(enable), Subsystem3/2(enable)

== system system_integration_v3/integration_v1/GA_main/coefficent_array/output_selector ==
  chose_port : Inport
  In2 : Inport  Port=2
  In3 : Inport  Port=3
  In4 : Inport  Port=4
  In5 : Inport  Port=5
  Multiport Switch : MultiPortSwitch  Inputs=4  SaturateOnIntegerOverflow=off  InputSameDT=off
  Switch : Switch  Criteria=u2 > Threshold  SaturateOnIntegerOverflow=off  InputSameDT=off
  Switch1 : Switch  Criteria=u2 > Threshold  SaturateOnIntegerOverflow=off  InputSameDT=off
  default_value : Constant  OutDataTypeStr=fixdt(0,4,0)  SampleTime=Ts
  ensure_correct_output : Constant  Value=0  OutDataTypeStr=fixdt(0,1,0)  SampleTime=Ts
  Out1 : Outport
  wires:
  chose_port/1 -> Switch1/1, Switch/2, Switch1/2
  In2/1 -> Multiport Switch/2
  default_value/1 -> Switch1/3
  In4/1 -> Multiport Switch/4
  Multiport Switch/1 -> Switch/1
  Switch1/1 -> Multiport Switch/1
  In3/1 -> Multiport Switch/3
  ensure_correct_output/1 -> Switch/3
  Switch/1 -> Out1/1
  In5/1 -> Multiport Switch/5

== system system_integration_v3/integration_v1/GA_main/coefficent_array/swap_counter ==
  In1 : Inport
  In2 : Inport  Port=2
  Add : Sum  OutDataTypeStr=fixdt(0,4,0)  AccumDataTypeStr=fixdt(0,4,0)
  Constant18 : Constant  OutDataTypeStr=fixdt(0,4,0)  SampleTime=Ts
  Constant19 : Constant  Value=0  OutDataTypeStr=fixdt(0,4,0)  SampleTime=Ts
  Constant20 : Constant  Value=0  OutDataTypeStr=fixdt(0,4,0)  SampleTime=Ts
  Delay : Delay  DelayLength=1  InitialCondition=0  SampleTime=Ts
  Switch : Switch  Criteria=u2 > Threshold  OutDataTypeStr=fixdt(0,4,0)  SaturateOnIntegerOverflow=off  InputSameDT=off
  Switch8 : Switch  Criteria=u2 > Threshold  OutDataTypeStr=fixdt(0,4,0)  SaturateOnIntegerOverflow=off  InputSameDT=off
  Out1 : Outport
  wires:
  Constant19/1 -> Switch/3
  Switch8/1 -> Add/2
  Switch/1 -> Add/1
  Delay/1 -> Out1/1, Switch8/3
  In2/1 -> Switch8/2
  Add/1 -> Delay/1
  Constant20/1 -> Switch8/1
  Constant18/1 -> Switch/1
  In1/1 -> Switch/2

== system system_integration_v3/integration_v1/GA_main/coefficent_array/swap_counter1 ==
  In1 : Inport
  In2 : Inport  Port=2
  Add : Sum  OutDataTypeStr=fixdt(0,4,0)  AccumDataTypeStr=fixdt(0,4,0)
  Constant18 : Constant  OutDataTypeStr=fixdt(0,4,0)  SampleTime=Ts
  Constant19 : Constant  Value=0  OutDataTypeStr=fixdt(0,4,0)  SampleTime=Ts
  Constant20 : Constant  OutDataTypeStr=fixdt(0,4,0)  SampleTime=Ts
  Delay : Delay  DelayLength=1  InitialCondition=0  SampleTime=Ts
  Switch : Switch  Criteria=u2 > Threshold  OutDataTypeStr=fixdt(0,4,0)  SaturateOnIntegerOverflow=off  InputSameDT=off
  Switch8 : Switch  Criteria=u2 > Threshold  OutDataTypeStr=fixdt(0,4,0)  SaturateOnIntegerOverflow=off  InputSameDT=off
  Out1 : Outport
  wires:
  Constant19/1 -> Switch/3
  Switch8/1 -> Add/2
  Switch/1 -> Add/1
  Delay/1 -> Out1/1, Switch8/3
  In2/1 -> Switch8/2
  Add/1 -> Delay/1
  Constant20/1 -> Switch8/1
  Constant18/1 -> Switch/1
  In1/1 -> Switch/2

== system system_integration_v3/integration_v1/GA_main/coefficent_array1/individual1 ==
  reg_in : Inport
  reg_in1 : Inport  Port=2
  reg_in2 : Inport  Port=3
  reg_in3 : Inport  Port=4
  reg_in4 : Inport  Port=5
  reg_in5 : Inport  Port=6
  reg_in6 : Inport  Port=7
  enable : Inport  Port=8
  Subsystem : Subsystem
  Subsystem1 : Subsystem
  Subsystem2 : Subsystem
  Subsystem3 : Subsystem
  Subsystem4 : Subsystem
  Subsystem5 : Subsystem
  Subsystem6 : Subsystem
  score : Outport
  a2 : Outport  Port=2
  a3 : Outport  Port=3
  a4 : Outport  Port=4
  b2 : Outport  Port=5
  b3 : Outport  Port=6
  b4 : Outport  Port=7
  wires:
  reg_in6/1 -> Subsystem6/1(reg_in)
  Subsystem6/1(reg_out) -> b4/1
  reg_in5/1 -> Subsystem5/1(reg_in)
  reg_in4/1 -> Subsystem4/1(reg_in)
  Subsystem5/1(reg_out) -> b3/1
  reg_in3/1 -> Subsystem3/1(reg_in)
  reg_in2/1 -> Subsystem2/1(reg_in)
  reg_in1/1 -> Subsystem1/1(reg_in)
  Subsystem/1(reg_out) -> score/1
  reg_in/1 -> Subsystem/1(reg_in)
  Subsystem1/1(reg_out) -> a2/1
  Subsystem3/1(reg_out) -> a4/1
  Subsystem4/1(reg_out) -> b2/1
  Subsystem2/1(reg_out) -> a3/1
  enable/1 -> Subsystem/2(enable), Subsystem1/2(enable), Subsystem2/2(enable), Subsystem6/2(enable), Subsystem5/2(enable), Subsystem4/2(enable), Subsystem3/2(enable)

== system system_integration_v3/integration_v1/GA_main/coefficent_array1/individual2 ==
  reg_in : Inport
  reg_in1 : Inport  Port=2
  reg_in2 : Inport  Port=3
  reg_in3 : Inport  Port=4
  reg_in4 : Inport  Port=5
  reg_in5 : Inport  Port=6
  reg_in6 : Inport  Port=7
  enable : Inport  Port=8
  Subsystem : Subsystem
  Subsystem1 : Subsystem
  Subsystem2 : Subsystem
  Subsystem3 : Subsystem
  Subsystem4 : Subsystem
  Subsystem5 : Subsystem
  Subsystem6 : Subsystem
  score : Outport
  a2 : Outport  Port=2
  a3 : Outport  Port=3
  a4 : Outport  Port=4
  b2 : Outport  Port=5
  b3 : Outport  Port=6
  b4 : Outport  Port=7
  wires:
  enable/1 -> Subsystem3/2(enable), Subsystem4/2(enable), Subsystem5/2(enable), Subsystem6/2(enable), Subsystem2/2(enable), Subsystem1/2(enable), Subsystem/2(enable)
  Subsystem2/1(reg_out) -> a3/1
  Subsystem4/1(reg_out) -> b2/1
  Subsystem3/1(reg_out) -> a4/1
  Subsystem1/1(reg_out) -> a2/1
  reg_in/1 -> Subsystem/1(reg_in)
  Subsystem/1(reg_out) -> score/1
  reg_in1/1 -> Subsystem1/1(reg_in)
  reg_in2/1 -> Subsystem2/1(reg_in)
  reg_in3/1 -> Subsystem3/1(reg_in)
  Subsystem5/1(reg_out) -> b3/1
  reg_in4/1 -> Subsystem4/1(reg_in)
  reg_in5/1 -> Subsystem5/1(reg_in)
  Subsystem6/1(reg_out) -> b4/1
  reg_in6/1 -> Subsystem6/1(reg_in)

== system system_integration_v3/integration_v1/GA_main/coefficent_array1/individual3 ==
  reg_in : Inport
  reg_in1 : Inport  Port=2
  reg_in2 : Inport  Port=3
  reg_in3 : Inport  Port=4
  reg_in4 : Inport  Port=5
  reg_in5 : Inport  Port=6
  reg_in6 : Inport  Port=7
  enable : Inport  Port=8
  Subsystem : Subsystem
  Subsystem1 : Subsystem
  Subsystem2 : Subsystem
  Subsystem3 : Subsystem
  Subsystem4 : Subsystem
  Subsystem5 : Subsystem
  Subsystem6 : Subsystem
  score : Outport
  a2 : Outport  Port=2
  a3 : Outport  Port=3
  a4 : Outport  Port=4
  b2 : Outport  Port=5
  b3 : Outport  Port=6
  b4 : Outport  Port=7
  wires:
  reg_in6/1 -> Subsystem6/1(reg_in)
  Subsystem6/1(reg_out) -> b4/1
  reg_in5/1 -> Subsystem5/1(reg_in)
  reg_in4/1 -> Subsystem4/1(reg_in)
  Subsystem5/1(reg_out) -> b3/1
  reg_in3/1 -> Subsystem3/1(reg_in)
  reg_in2/1 -> Subsystem2/1(reg_in)
  reg_in1/1 -> Subsystem1/1(reg_in)
  Subsystem/1(reg_out) -> score/1
  reg_in/1 -> Subsystem/1(reg_in)
  Subsystem1/1(reg_out) -> a2/1
  Subsystem3/1(reg_out) -> a4/1
  Subsystem4/1(reg_out) -> b2/1
  Subsystem2/1(reg_out) -> a3/1
  enable/1 -> Subsystem/2(enable), Subsystem1/2(enable), Subsystem2/2(enable), Subsystem6/2(enable), Subsystem5/2(enable), Subsystem4/2(enable), Subsystem3/2(enable)

== system system_integration_v3/integration_v1/GA_main/coefficent_array1/individual4 ==
  reg_in : Inport
  reg_in1 : Inport  Port=2
  reg_in2 : Inport  Port=3
  reg_in3 : Inport  Port=4
  reg_in4 : Inport  Port=5
  reg_in5 : Inport  Port=6
  reg_in6 : Inport  Port=7
  enable : Inport  Port=8
  Subsystem : Subsystem
  Subsystem1 : Subsystem
  Subsystem2 : Subsystem
  Subsystem3 : Subsystem
  Subsystem4 : Subsystem
  Subsystem5 : Subsystem
  Subsystem6 : Subsystem
  score : Outport
  a2 : Outport  Port=2
  a3 : Outport  Port=3
  a4 : Outport  Port=4
  b2 : Outport  Port=5
  b3 : Outport  Port=6
  b4 : Outport  Port=7
  wires:
  enable/1 -> Subsystem3/2(enable), Subsystem4/2(enable), Subsystem5/2(enable), Subsystem6/2(enable), Subsystem2/2(enable), Subsystem1/2(enable), Subsystem/2(enable)
  Subsystem2/1(reg_out) -> a3/1
  Subsystem4/1(reg_out) -> b2/1
  Subsystem3/1(reg_out) -> a4/1
  Subsystem1/1(reg_out) -> a2/1
  reg_in/1 -> Subsystem/1(reg_in)
  Subsystem/1(reg_out) -> score/1
  reg_in1/1 -> Subsystem1/1(reg_in)
  reg_in2/1 -> Subsystem2/1(reg_in)
  reg_in3/1 -> Subsystem3/1(reg_in)
  Subsystem5/1(reg_out) -> b3/1
  reg_in4/1 -> Subsystem4/1(reg_in)
  reg_in5/1 -> Subsystem5/1(reg_in)
  Subsystem6/1(reg_out) -> b4/1
  reg_in6/1 -> Subsystem6/1(reg_in)

== system system_integration_v3/integration_v1/GA_main/coefficent_array1/output_selector ==
  chose_port : Inport
  In2 : Inport  Port=2
  In3 : Inport  Port=3
  In4 : Inport  Port=4
  In5 : Inport  Port=5
  Multiport Switch : MultiPortSwitch  Inputs=4  SaturateOnIntegerOverflow=off  InputSameDT=off
  Switch : Switch  Criteria=u2 > Threshold  SaturateOnIntegerOverflow=off  InputSameDT=off
  Switch1 : Switch  Criteria=u2 > Threshold  SaturateOnIntegerOverflow=off  InputSameDT=off
  default_value : Constant  OutDataTypeStr=fixdt(0,4,0)  SampleTime=Ts
  ensure_correct_output : Constant  Value=0  OutDataTypeStr=fixdt(0,1,0)  SampleTime=Ts
  Out1 : Outport
  wires:
  In5/1 -> Multiport Switch/5
  Switch/1 -> Out1/1
  ensure_correct_output/1 -> Switch/3
  In3/1 -> Multiport Switch/3
  Switch1/1 -> Multiport Switch/1
  Multiport Switch/1 -> Switch/1
  In4/1 -> Multiport Switch/4
  default_value/1 -> Switch1/3
  In2/1 -> Multiport Switch/2
  chose_port/1 -> Switch1/2, Switch/2, Switch1/1

== system system_integration_v3/integration_v1/GA_main/coefficent_array1/swap_counter ==
  In1 : Inport
  In2 : Inport  Port=2
  Add : Sum  OutDataTypeStr=fixdt(0,4,0)  AccumDataTypeStr=fixdt(0,4,0)
  Constant18 : Constant  OutDataTypeStr=fixdt(0,4,0)  SampleTime=Ts
  Constant19 : Constant  Value=0  OutDataTypeStr=fixdt(0,4,0)  SampleTime=Ts
  Constant20 : Constant  Value=0  OutDataTypeStr=fixdt(0,4,0)  SampleTime=Ts
  Delay : Delay  DelayLength=1  InitialCondition=0  SampleTime=Ts
  Switch : Switch  Criteria=u2 > Threshold  OutDataTypeStr=fixdt(0,4,0)  SaturateOnIntegerOverflow=off  InputSameDT=off
  Switch8 : Switch  Criteria=u2 > Threshold  OutDataTypeStr=fixdt(0,4,0)  SaturateOnIntegerOverflow=off  InputSameDT=off
  Out1 : Outport
  wires:
  In1/1 -> Switch/2
  Constant18/1 -> Switch/1
  Constant20/1 -> Switch8/1
  Add/1 -> Delay/1
  In2/1 -> Switch8/2
  Delay/1 -> Switch8/3, Out1/1
  Switch/1 -> Add/1
  Switch8/1 -> Add/2
  Constant19/1 -> Switch/3

== system system_integration_v3/integration_v1/GA_main/coefficent_array1/swap_counter1 ==
  In1 : Inport
  In2 : Inport  Port=2
  Add : Sum  OutDataTypeStr=fixdt(0,4,0)  AccumDataTypeStr=fixdt(0,4,0)
  Constant18 : Constant  OutDataTypeStr=fixdt(0,4,0)  SampleTime=Ts
  Constant19 : Constant  Value=0  OutDataTypeStr=fixdt(0,4,0)  SampleTime=Ts
  Constant20 : Constant  OutDataTypeStr=fixdt(0,4,0)  SampleTime=Ts
  Delay : Delay  DelayLength=1  InitialCondition=0  SampleTime=Ts
  Switch : Switch  Criteria=u2 > Threshold  OutDataTypeStr=fixdt(0,4,0)  SaturateOnIntegerOverflow=off  InputSameDT=off
  Switch8 : Switch  Criteria=u2 > Threshold  OutDataTypeStr=fixdt(0,4,0)  SaturateOnIntegerOverflow=off  InputSameDT=off
  Out1 : Outport
  wires:
  In1/1 -> Switch/2
  Constant18/1 -> Switch/1
  Constant20/1 -> Switch8/1
  Add/1 -> Delay/1
  In2/1 -> Switch8/2
  Delay/1 -> Switch8/3, Out1/1
  Switch/1 -> Add/1
  Switch8/1 -> Add/2
  Constant19/1 -> Switch/3

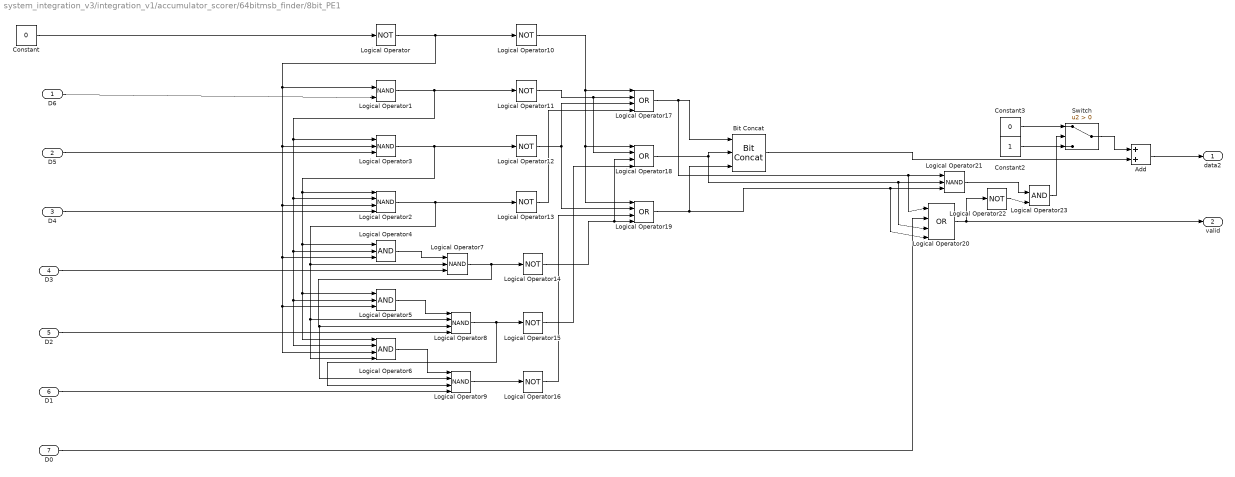
== system system_integration_v3/integration_v1/accumulator_scorer/64bitmsb_finder/8bit_PE1 ==
  D6 : Inport
  D5 : Inport  Port=2
  D4 : Inport  Port=3
  D3 : Inport  Port=4
  D2 : Inport  Port=5
  D1 : Inport  Port=6
  D0 : Inport  Port=7
  Add : Sum
  Bit Concat : hdlsllib/Logic and Bit Operations/Bit Concat  numInputs=3
  Constant : Constant  Value=0  OutDataTypeStr=boolean  SampleTime=Ts
  Constant2 : Constant  OutDataTypeStr=fixdt(0,4,0)  SampleTime=Ts
  Constant3 : Constant  Value=0  OutDataTypeStr=fixdt(0,4,0)  SampleTime=Ts
  Logical Operator{,10..16,22} (9 alike) : Logic  Operator=NOT  IconShape=distinctive  AllPortsSameDT=off  OutDataTypeStr=boolean
  Logical Operator1 : Logic  Operator=NAND  IconShape=distinctive  AllPortsSameDT=off  OutDataTypeStr=boolean
  Logical Operator{17..20} (4 alike) : Logic  Operator=OR  Inputs=4  IconShape=distinctive  AllPortsSameDT=off  OutDataTypeStr=boolean
  Logical Operator2 : Logic  Operator=NAND  Inputs=4  IconShape=distinctive  AllPortsSameDT=off  OutDataTypeStr=boolean
  Logical Operator21 : Logic  Operator=NAND  Inputs=3  IconShape=distinctive  AllPortsSameDT=off  OutDataTypeStr=boolean
  Logical Operator23 : Logic  IconShape=distinctive  AllPortsSameDT=off  OutDataTypeStr=boolean
  Logical Operator3 : Logic  Operator=NAND  Inputs=3  IconShape=distinctive  AllPortsSameDT=off  OutDataTypeStr=boolean
  Logical Operator4 : Logic  Inputs=3  IconShape=distinctive  AllPortsSameDT=off  OutDataTypeStr=boolean
  Logical Operator5 : Logic  Inputs=3  IconShape=distinctive  AllPortsSameDT=off  OutDataTypeStr=boolean
  Logical Operator6 : Logic  Inputs=4  IconShape=distinctive  AllPortsSameDT=off  OutDataTypeStr=boolean
  Logical Operator7 : Logic  Operator=NAND  Inputs=3  IconShape=distinctive  AllPortsSameDT=off  OutDataTypeStr=boolean
  Logical Operator8 : Logic  Operator=NAND  Inputs=4  IconShape=distinctive  AllPortsSameDT=off  OutDataTypeStr=boolean
  Logical Operator9 : Logic  Operator=NAND  Inputs=4  IconShape=distinctive  AllPortsSameDT=off  OutDataTypeStr=boolean
  Switch : Switch  Criteria=u2 > Threshold  SaturateOnIntegerOverflow=off  InputSameDT=off  OutDataTypeStr=Inherit: Same as first input
  data2 : Outport
  valid : Outport  Port=2
  wires:
  Logical Operator22/1 -> Logical Operator23/2
  Logical Operator23/1 -> Switch/2
  Logical Operator21/1 -> Logical Operator23/1
  Constant2/1 -> Switch/3
  Bit Concat/1 -> Add/2
  Add/1 -> data2/1
  Constant3/1 -> Switch/1
  Switch/1 -> Add/1
  Logical Operator20/1 -> Logical Operator22/1, valid/1
  D0/1 -> Logical Operator20/2
  Logical Operator9/1 -> Logical Operator16/1
  Logical Operator16/1 -> Logical Operator19/3
  Logical Operator11/1 -> Logical Operator17/2, Logical Operator18/2
  D6/1 -> Logical Operator1/2
  Logical Operator6/1 -> Logical Operator9/1
  Logical Operator8/1 -> Logical Operator15/1, Logical Operator9/3
  Logical Operator4/1 -> Logical Operator7/1
  D1/1 -> Logical Operator9/4
  Logical Operator5/1 -> Logical Operator8/1
  D2/1 -> Logical Operator8/4
  Logical Operator17/1 -> Bit Concat/1, Logical Operator21/1, Logical Operator20/1
  D5/1 -> Logical Operator3/3
  Logical Operator14/1 -> Logical Operator19/4, Logical Operator18/3
  Logical Operator10/1 -> Logical Operator17/1, Logical Operator18/1, Logical Operator19/1
  Logical Operator15/1 -> Logical Operator18/4
  Constant/1 -> Logical Operator/1
  D3/1 -> Logical Operator7/3
  Logical Operator19/1 -> Bit Concat/3, Logical Operator21/3, Logical Operator20/4
  Logical Operator12/1 -> Logical Operator19/2, Logical Operator17/3
  Logical Operator/1 -> Logical Operator10/1, Logical Operator3/2, Logical Operator4/3, Logical Operator5/3, Logical Operator6/3, Logical Operator2/3, Logical Operator1/1
  Logical Operator7/1 -> Logical Operator14/1, Logical Operator8/3, Logical Operator9/2
  D4/1 -> Logical Operator2/4
  Logical Operator13/1 -> Logical Operator17/4
  Logical Operator3/1 -> Logical Operator12/1, Logical Operator4/1, Logical Operator5/1, Logical Operator6/1, Logical Operator2/1
  Logical Operator18/1 -> Logical Operator21/2, Logical Operator20/3, Bit Concat/2
  Logical Operator2/1 -> Logical Operator13/1, Logical Operator7/2, Logical Operator8/2, Logical Operator6/4
  Logical Operator1/1 -> Logical Operator11/1, Logical Operator3/1, Logical Operator2/2, Logical Operator5/2, Logical Operator6/2, Logical Operator4/2
